simulink model "P4p3"  (R2014a)
settings: Solver=ode1  StartTime=0.0  StopTime=inf  FixedStep=0.02  RelTol=1e-3
PostLoadFcn:
  | qc_set_target_type(getConfigSet(bdroot, 'QUARC Default Target Configuration'));
values from neighbouring files (symbols this model uses):
  A_est = [0 1 0 0 0 0 ... (first row only)    [P4p2_init.m]    (also in P4p3_init.m)
  B_est = [0,0 ... (first row only)    [P4p2_init.m]    (also in P4p3_init.m)
  C_est = [1 0 0 0 0 0 ... (first row only)    [P4p2_init.m]    (also in P4p3_init.m = [0 0 0 0 0 0)
  K_LQR = lqr(A_PI,B_PI,Q_est,R_est)    [P4p2_init.m]    (also in P4p3_init.m)
  L_est = abs(place(A_est', C_est', L_poles)')    [P4p2_init.m]    (also in P4p3_init.m)
  P_LQR = inv(C_P*inv(B_P*K_LQR_P-A_P)*B_P)    [P4p2_init.m]    (also in P4p3_init.m)
undefined symbols (not defined in the file or in its folder): HIL, Joystick_gain_x, Joystick_gain_y, qc_get_step_size
libraries: simulink_extras x6, quarc_library x4
settings Model: SimulationMode=external  ExtModeTrigDuration=5000  Creator=Rchan  LastModifiedBy=evenwa
settings SolverCC: PositivePriorityOrder=on
settings DataIOCC: SignalLoggingSaveFormat=ModelDataLogs
settings OptimizationCC: ExpressionDepthLimit=2147483647  InitFltsAndDblsToZero=on
settings DebuggingCC: SaveWithParameterizedLinksMsg=none  UnderspecifiedInitializationDetection=Classic  MultiTaskDSMMsg=warning  MultiTaskCondExecSysMsg=none  FcnCallInpInsideContextMsg=UseLocalSettings  StateNameClashWarn=warning
settings RTWCC: SystemTargetFile=quarc_win64.tlc  TemplateMakefile=quarc_default_tmf  Description=QUARC Win64 Target  ProcessScript=quarc_win64_make_rtw_hook
settings STFCustomTargetCC: CPPClassGenCompliant=on
settings GRTTargetCC: ParMdlRefBuildCompliant=off  CompOptLevelCompliant=off  CombineOutputUpdateFcns=off  MatFileLogging=off  GRTInterface=on  ExtMode=on  ExtModeMexFile=quarc_comm

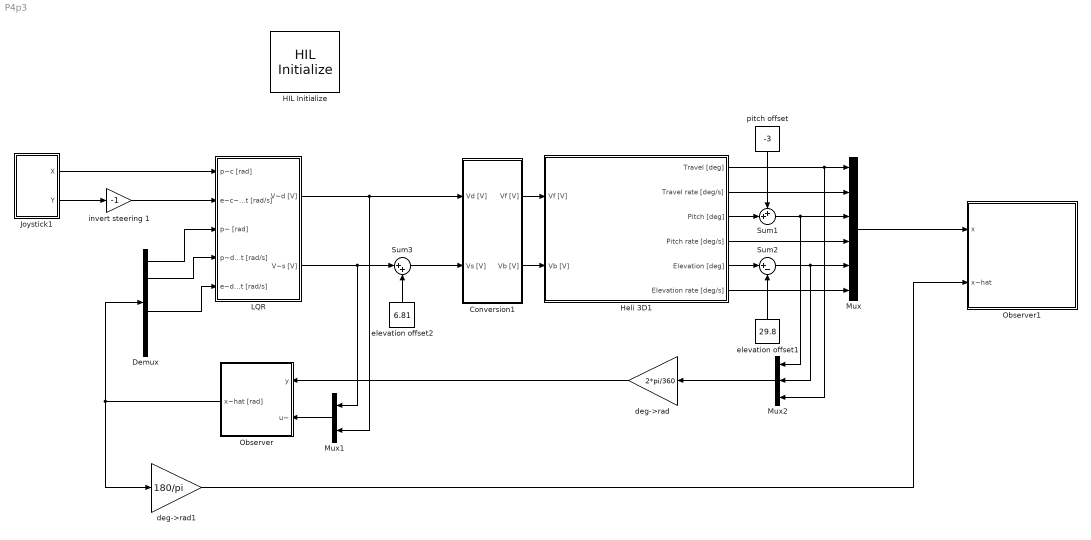
== system P4p3 ==
  Conversion1 : Subsystem
  Demux : Demux  Outputs=6
  HIL Initialize : quarc_library/Data Acquisition/Generic/Configuration/HIL Initialize  Priority=-99  object_name=HIL-1  board_type=q8_usb  board_number=0  board_options=update_rate=normal;decimation=1  exclusive=off  active=off  hardware_clocks=[0:2]  clock_modes=[]  initial_clock_frequencies=[]  set_clock_params_at_start=off  set_clock_params_at_switch_in=off  set_clock_frequencies_at_start=off  set_clock_frequencies_at_switch_in=off  analog_input_channels=[0:7]  analog_input_maximums=10  analog_input_minimums=-10  set_analog_input_params_at_start=on  set_analog_input_params_at_switch_in=off  analog_output_channels=[0:7]  analog_output_maximums=10  analog_output_minimums=-10  initial_analog_outputs=[0]  final_analog_outputs=[0]  watchdog_analog_outputs=0  set_analog_output_params_at_start=on  set_analog_output_params_at_switch_in=off  set_analog_outputs_at_start=on  set_analog_outputs_at_switch_in=off  set_analog_outputs_at_terminate=on  set_analog_outputs_at_switch_out=off  set_analog_outputs_on_watchdog=off  digital_input_channels=[]  digital_output_channels=[]  digital_output_configuration=[]  initial_digital_outputs=[1]  final_digital_outputs=[1]  watchdog_digital_outputs=[1]  set_digital_output_params_at_start=off  set_digital_output_params_at_switch_in=off  set_digital_outputs_at_start=on  set_digital_outputs_at_switch_in=off  set_digital_outputs_at_terminate=on  set_digital_outputs_at_switch_out=off  set_digital_outputs_on_watchdog=off  encoder_channels=[0:7]  quadrature=[4]  encoder_filter_frequency=[]  initial_encoder_counts=[0]  set_encoder_params_at_start=on  set_encoder_params_at_switch_in=off  set_encoder_counts_at_start=on  set_encoder_counts_at_switch_in=off  pwm_channels=[0:7]  pwm_modes=0  pwm_frequency=99.532799999999995e6/4095  pwm_configuration=[0]  pwm_alignment=[0]  pwm_polarity=[1]  pwm_leading_deadband=[0]  pwm_trailing_deadband=[0]  initial_pwm_outputs=[0]  final_pwm_outputs=[0]  watchdog_pwm_outputs=[0]  set_pwm_params_at_start=on  set_pwm_params_at_switch_in=off  set_pwm_outputs_at_start=on  set_pwm_outputs_at_switch_in=off  set_pwm_outputs_at_terminate=on  set_pwm_outputs_at_switch_out=off  set_pwm_outputs_on_watchdog=off  other_output_channels=[]  initial_other_outputs=[]  final_other_outputs=[]  watchdog_other_outputs=[]  set_other_outputs_at_start=off  set_other_outputs_at_switch_in=off  set_other_outputs_at_terminate=off  set_other_outputs_at_switch_out=off  set_other_outputs_on_watchdog=off
  Heli 3D1 : Subsystem
  Joystick1 : Subsystem
  LQR : Subsystem  ClipboardFcn=set_param(gcb, 'BackgrounColor', 'red');
  Mux : Mux  Inputs=6
  Mux1 : Mux  Inputs=2
  Mux2 : Mux  Inputs=3
  Observer : Subsystem  ClipboardFcn=set_param(gcb, 'BackgrounColor', 'red');
  Observer1 : Subsystem  ClipboardFcn=set_param(gcb, 'BackgrounColor', 'red');
  Sum1 : Sum  Inputs=++|
  Sum2 : Sum  Inputs=|+-
  Sum3 : Sum  Inputs=|++
  deg->rad : Gain  Gain=2*pi/360
  deg->rad1 : Gain  Gain=180/pi
  elevation offset1 : Constant  Value=29.8
  elevation offset2 : Constant  Value=6.81
  invert steering 1 : Gain  Gain=-1
  pitch offset : Constant  Value=-3
  wires:
  Conversion1/2(Vb [V]) -> Heli 3D1/2(Vb [V])
  Conversion1/1(Vf [V]) -> Heli 3D1/1(Vf [V])
  Heli 3D1/3(Pitch [deg]) -> Sum1/2
  elevation offset1/1 -> Sum2/2
  Heli 3D1/5(Elevation [deg]) -> Sum2/1
  pitch offset/1 -> Sum1/1
  LQR/1(V~d [V]) -> Mux1/2, Conversion1/1(Vd [V])
  LQR/2(V~s [V]) -> Mux1/1, Sum3/1
  deg->rad/1 -> Observer/1(y)
  Demux/1 -> LQR/3(p~ [rad])
  Demux/2 -> LQR/4(p~dot [rad/s])
  Demux/4 -> LQR/5(e~dot [rad/s])
  Observer/1(x~hat [rad]) -> Demux/1, deg->rad1/1
  elevation offset2/1 -> Sum3/2
  Sum3/1 -> Conversion1/2(Vs [V])
  invert steering 1/1 -> LQR/2(e~c~dot [rad/s])
  Joystick1/2(Y) -> invert steering 1/1
  Heli 3D1/1(Travel [deg]) -> Mux2/3, Mux/1
  Sum1/1 -> Mux/3, Mux2/1
  Sum2/1 -> Mux/5, Mux2/2
  Joystick1/1(X) -> LQR/1(p~c [rad])
  Mux1/1 -> Observer/2(u~)
  Mux2/1 -> deg->rad/1
  Heli 3D1/2(Travel rate [deg/s]) -> Mux/2
  Heli 3D1/4(Pitch rate [deg/s]) -> Mux/4
  Heli 3D1/6(Elevation rate [deg/s]) -> Mux/6
  Mux/1 -> Observer1/1(x)
  deg->rad1/1 -> Observer1/2(x~hat)

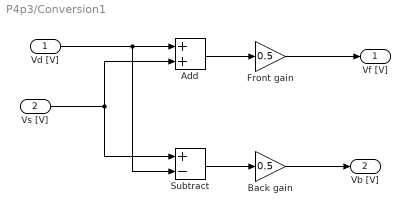
== system P4p3/Conversion1 ==
  Vd [V] : Inport
  Vs [V] : Inport  Port=2
  Add : Sum
  Back gain : Gain  Gain=0.5
  Front gain : Gain  Gain=0.5
  Subtract : Sum  Inputs=+-
  Vf [V] : Outport
  Vb [V] : Outport  Port=2
  wires:
  Vd [V]/1 -> Subtract/2, Add/1
  Vs [V]/1 -> Subtract/1, Add/2
  Subtract/1 -> Back gain/1
  Back gain/1 -> Vb [V]/1
  Add/1 -> Front gain/1
  Front gain/1 -> Vf [V]/1

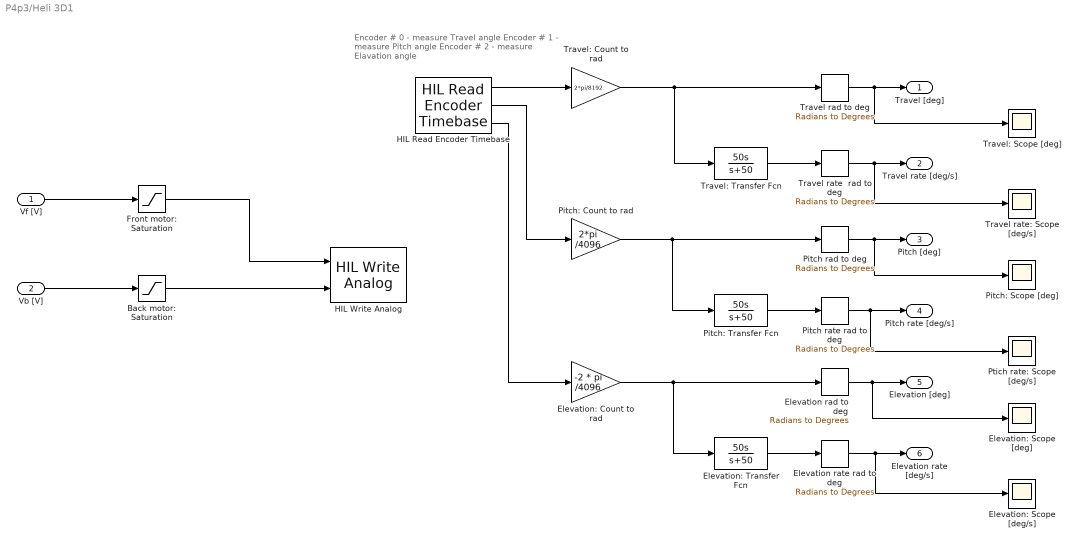
== system P4p3/Heli 3D1 ==
  note: Encoder # 0 - measure Travel angle
      | Encoder # 1 - measure Pitch angle
      | Encoder # 2 - measure Elavation angle
  Vf [V] : Inport
  Vb [V] : Inport  Port=2
  Back motor: Saturation : Saturate  UpperLimit=5  LowerLimit=-5
  Elevation rad to deg : simulink_extras/Transformations/Radians to Degrees
  Elevation rate rad to deg : simulink_extras/Transformations/Radians to Degrees
  Elevation: Count to rad : Gain  Gain=-2 * pi /4096
  Elevation: Scope [deg/s] : Scope
      settings: YMax=25  SaveName=ScopeData13
  Elevation: Scope [deg] : Scope
      settings: YMin=-0  YMax=45  SaveName=ScopeData12
  Elevation: Transfer Fcn : TransferFcn  Numerator=[50 0]  Denominator=[1 50]
  Front motor: Saturation : Saturate  UpperLimit=5  LowerLimit=-5
  HIL Read Encoder Timebase : quarc_library/Data Acquisition/Generic/Timebases/HIL Read Encoder Timebase  object_name=HIL-1  clock=0  channels=[0:2]  samples_in_buffer=max(ceil(1/qc_get_step_size), 1)  active=on  vector_output=off  data_type_mode=Inherit via back propagation  data_type=double
  HIL Write Analog : quarc_library/Data Acquisition/Generic/Immediate I//O/HIL Write Analog  object_name=HIL-1  channels=[0:1]  sample_time=-1  active=off  vector_input=off
  Pitch rad to deg : simulink_extras/Transformations/Radians to Degrees
  Pitch rate rad to deg : simulink_extras/Transformations/Radians to Degrees
  Pitch: Count to rad : Gain  Gain=2*pi /4096
  Pitch: Scope [deg] : Scope
      settings: YMin=-45  YMax=40  SaveName=ScopeData10
  Pitch: Transfer Fcn : TransferFcn  Numerator=[50 0]  Denominator=[1 50]
  Ptich rate: Scope [deg/s] : Scope
      settings: YMin=-15  YMax=15  SaveName=ScopeData11
  Travel rad to deg : simulink_extras/Transformations/Radians to Degrees
  Travel rate  rad to deg : simulink_extras/Transformations/Radians to Degrees
  Travel rate: Scope [deg/s] : Scope
      settings: YMin=-15  YMax=15  SaveName=ScopeData9
  Travel: Count to rad : Gain  Gain=2*pi/8192
  Travel: Scope [deg] : Scope
      settings: YMin=-107.5  YMax=-72.5  SaveName=ScopeData8
  Travel: Transfer Fcn : TransferFcn  Numerator=[50 0]  Denominator=[1 50]
  Travel [deg] : Outport
  Travel rate [deg/s] : Outport  Port=2
  Pitch [deg] : Outport  Port=3
  Pitch rate [deg/s] : Outport  Port=4
  Elevation [deg] : Outport  Port=5
  Elevation rate [deg/s] : Outport  Port=6
  wires:
  HIL Read Encoder Timebase/1 -> Travel: Count to rad/1
  HIL Read Encoder Timebase/2 -> Pitch: Count to rad/1
  HIL Read Encoder Timebase/3 -> Elevation: Count to rad/1
  Travel: Count to rad/1 -> Travel: Transfer Fcn/1, Travel rad to deg/1
  Travel: Transfer Fcn/1 -> Travel rate  rad to deg/1
  Pitch: Count to rad/1 -> Pitch: Transfer Fcn/1, Pitch rad to deg/1
  Pitch: Transfer Fcn/1 -> Pitch rate rad to deg/1
  Elevation: Count to rad/1 -> Elevation: Transfer Fcn/1, Elevation rad to deg/1
  Elevation: Transfer Fcn/1 -> Elevation rate rad to deg/1
  Travel rad to deg/1 -> Travel: Scope [deg]/1, Travel [deg]/1
  Travel rate  rad to deg/1 -> Travel rate: Scope [deg/s]/1, Travel rate [deg/s]/1
  Pitch rad to deg/1 -> Pitch: Scope [deg]/1, Pitch [deg]/1
  Pitch rate rad to deg/1 -> Ptich rate: Scope [deg/s]/1, Pitch rate [deg/s]/1
  Elevation rad to deg/1 -> Elevation: Scope [deg]/1, Elevation [deg]/1
  Elevation rate rad to deg/1 -> Elevation: Scope [deg/s]/1, Elevation rate [deg/s]/1
  Vf [V]/1 -> Front motor: Saturation/1
  Vb [V]/1 -> Back motor: Saturation/1
  Front motor: Saturation/1 -> HIL Write Analog/1
  Back motor: Saturation/1 -> HIL Write Analog/2

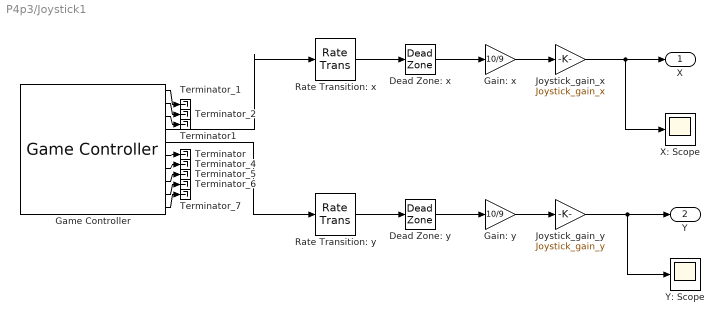
== system P4p3/Joystick1 ==
  Dead Zone: x : DeadZone  LowerValue=-0.1  UpperValue=0.1  SaturateOnIntegerOverflow=on
  Dead Zone: y : DeadZone  LowerValue=-0.1  UpperValue=0.1  SaturateOnIntegerOverflow=on
  Gain: x : Gain  Gain=10/9
  Gain: y : Gain  Gain=10/9
  Game Controller : quarc_library/Devices/Peripherals/Target/Game Controller  controller=1  buffer_size=12  deadzone=[]  saturation=[]  sample_time=max(qc_get_step_size, 0.01)  auto_center=off  enabled=on
  Joystick_gain_x : Gain  Gain=Joystick_gain_x
  Joystick_gain_y : Gain  Gain=Joystick_gain_y
  Rate Transition: x : RateTransition
  Rate Transition: y : RateTransition
  Terminator : Terminator
  Terminator1 : Terminator
  Terminator_{1..2,4..7} (6 alike) : Terminator
  X: Scope : Scope
      settings: YMin=-1  YMax=1  SaveName=ScopeData7
  Y: Scope : Scope
      settings: YMin=-10  YMax=10  SaveName=ScopeData5
  X : Outport
  Y : Outport  Port=2
  wires:
  Rate Transition: y/1 -> Dead Zone: y/1
  Rate Transition: x/1 -> Dead Zone: x/1
  Game Controller/5 -> Rate Transition: y/1
  Game Controller/4 -> Rate Transition: x/1
  Game Controller/1 -> Terminator_1/1
  Game Controller/2 -> Terminator_2/1
  Game Controller/7 -> Terminator_4/1
  Game Controller/8 -> Terminator_5/1
  Game Controller/9 -> Terminator_6/1
  Game Controller/10 -> Terminator_7/1
  Game Controller/3 -> Terminator1/1
  Game Controller/6 -> Terminator/1
  Dead Zone: x/1 -> Gain: x/1
  Dead Zone: y/1 -> Gain: y/1
  Gain: x/1 -> Joystick_gain_x/1
  Gain: y/1 -> Joystick_gain_y/1
  Joystick_gain_x/1 -> X/1, X: Scope/1
  Joystick_gain_y/1 -> Y: Scope/1, Y/1

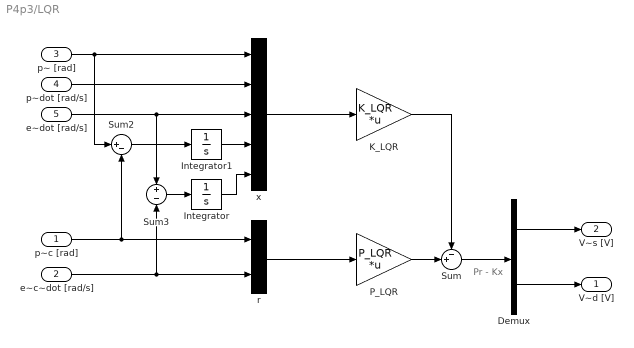
== system P4p3/LQR ==
  note: Pr - Kx
  p~c [rad] : Inport
  e~c~dot [rad/s] : Inport  Port=2
  p~ [rad] : Inport  Port=3
  p~dot [rad/s] : Inport  Port=4
  e~dot [rad/s] : Inport  Port=5
  Demux : Demux  Outputs=2
  Integrator : Integrator
  Integrator1 : Integrator
  K_LQR : Gain  Gain=K_LQR  Multiplication=Matrix(K*u)
  P_LQR : Gain  Gain=P_LQR  Multiplication=Matrix(K*u)
  Sum : Sum  Inputs=-+|
  Sum2 : Sum  Inputs=|+-
  Sum3 : Sum  Inputs=+-
  r : Concatenate
  x : Concatenate  NumInputs=5
  V~d [V] : Outport  InitialOutput=0
  V~s [V] : Outport  Port=2  InitialOutput=0
  wires:
  Demux/1 -> V~s [V]/1
  Demux/2 -> V~d [V]/1
  Sum/1 -> Demux/1
  x/1 -> K_LQR/1
  p~dot [rad/s]/1 -> x/2
  p~ [rad]/1 -> Sum2/1, x/1
  e~dot [rad/s]/1 -> x/3, Sum3/1
  e~c~dot [rad/s]/1 -> r/2, Sum3/2
  r/1 -> P_LQR/1
  p~c [rad]/1 -> r/1, Sum2/2
  P_LQR/1 -> Sum/2
  K_LQR/1 -> Sum/1
  Sum2/1 -> Integrator1/1
  Sum3/1 -> Integrator/1
  Integrator/1 -> x/5
  Integrator1/1 -> x/4

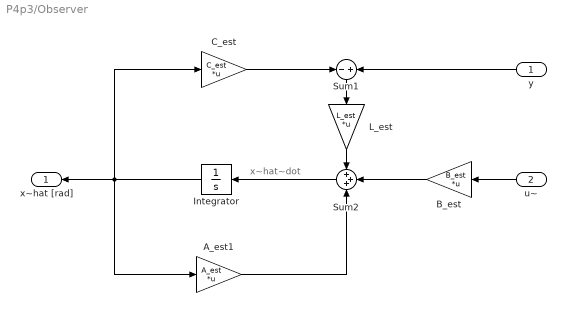
== system P4p3/Observer ==
  note: x~hat~dot
  y : Inport
  u~ : Inport  Port=2
  A_est1 : Gain  Gain=A_est  Multiplication=Matrix(K*u)
  B_est : Gain  Gain=B_est  Multiplication=Matrix(K*u)
  C_est : Gain  Gain=C_est  Multiplication=Matrix(K*u)
  Integrator : Integrator
  L_est : Gain  Gain=L_est  Multiplication=Matrix(K*u)
  Sum1 : Sum  Inputs=-+
  Sum2 : Sum  Inputs=+++
  x~hat [rad] : Outport  InitialOutput=0
  wires:
  Integrator/1 -> A_est1/1, C_est/1, x~hat [rad]/1
  u~/1 -> B_est/1
  y/1 -> Sum1/2
  B_est/1 -> Sum2/2
  Sum1/1 -> L_est/1
  L_est/1 -> Sum2/1
  Sum2/1 -> Integrator/1
  C_est/1 -> Sum1/1
  A_est1/1 -> Sum2/3

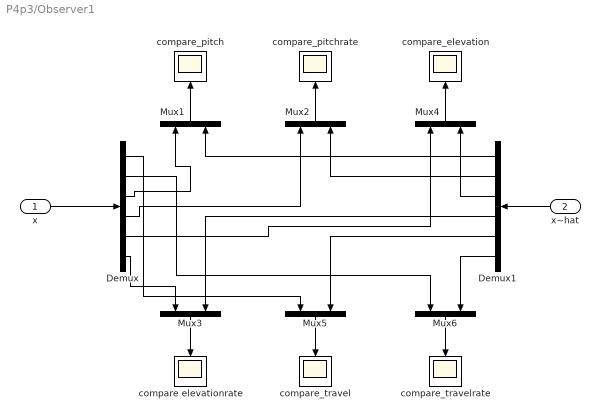
== system P4p3/Observer1 ==
  x : Inport
  x~hat : Inport  Port=2
  Demux : Demux  Outputs=6
  Demux1 : Demux  Outputs=6
  Mux{1..6} (6 alike) : Mux  Inputs=2
  compare elevationrate : Scope
      settings: YMin=-1.5  YMax=4.5  SaveName=ScopeData2
  compare_elevation : Scope
      settings: YMin=-4.4  YMax=-3.75  SaveName=ScopeData3
  compare_pitch : Scope
      settings: YMin=-8  YMax=3
  compare_pitchrate : Scope
  compare_travel : Scope
      settings: YMin=100  YMax=155  SaveName=ScopeData4
  compare_travelrate : Scope
      settings: YMin=0  YMax=7  SaveName=ScopeData6
  wires:
  x/1 -> Demux/1
  Mux1/1 -> compare_pitch/1
  Mux2/1 -> compare_pitchrate/1
  x~hat/1 -> Demux1/1
  Demux1/1 -> Mux1/2
  Demux1/2 -> Mux2/2
  Mux4/1 -> compare_elevation/1
  Demux1/3 -> Mux4/2
  Demux1/5 -> Mux5/2
  Mux5/1 -> compare_travel/1
  Mux3/1 -> compare elevationrate/1
  Demux1/4 -> Mux3/2
  Mux6/1 -> compare_travelrate/1
  Demux1/6 -> Mux6/2
  Demux/1 -> Mux5/1
  Demux/2 -> Mux6/1
  Demux/3 -> Mux1/1
  Demux/4 -> Mux2/1
  Demux/6 -> Mux3/1
  Demux/5 -> Mux4/1
